simulink model "Matrice_masse_manipulateur"  (R2022b)
settings: Solver=VariableStepAuto  StartTime=0.0  StopTime=10.0  RelTol=1e-3
undefined symbols (not defined in the file): l1, l2, m1, m2
settings Model: Creator=cheye  LastModifiedBy=cheye

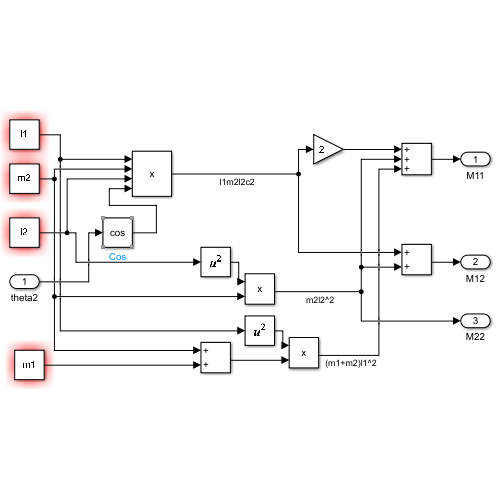
[thumbnail: Simulink's stored preview of the top-level diagram]
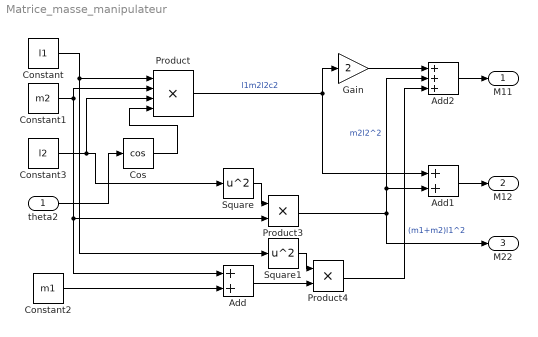
== system Matrice_masse_manipulateur ==
  theta2 : Inport
  Add : Sum
  Add1 : Sum
  Add2 : Sum  Inputs=+++
  Constant : Constant  Value=l1
  Constant1 : Constant  Value=m2
  Constant2 : Constant  Value=m1
  Constant3 : Constant  Value=l2
  Cos : Trigonometry  Operator=cos
  Gain : Gain  Gain=2
  Product : Product  Inputs=4
  Product3 : Product
  Product4 : Product
  Square : Math  Operator=square
  Square1 : Math  Operator=square
  M11 : Outport
  M12 : Outport  Port=2
  M22 : Outport  Port=3
  wires:
  Constant/1 -> Product/1, Square1/1
  Constant1/1 -> Product/2, Add/1, Product3/2
  Constant3/1 -> Product/3, Square/1
  Square/1 -> Product3/1
  Constant2/1 -> Add/2
  Square1/1 -> Product4/1
  Add/1 -> Product4/2
  Product/1 -> Add1/1, Gain/1  "l1m2l2c2"
  Gain/1 -> Add2/1
  Add2/1 -> M11/1
  Product3/1 -> M22/1, Add2/2, Add1/2  "m2l2^2"
  Add1/1 -> M12/1
  Product4/1 -> Add2/3  "(m1+m2)l1^2"
  theta2/1 -> Cos/1
  Cos/1 -> Product/4
